simulink model "verify_com_acceleration_computation"  (R2015a)
settings: Solver=ode45  StartTime=0.0  StopTime=1.2  RelTol=1e-3
undefined symbols (not defined in the file or in its folder): A_kalman_transverse, A_kalman_vertical, B_kalman_transverse, B_kalman_vertical, C_kalman_transverse, C_kalman_vertical, com_leg_motor, com_torso, Discrete, g, initial_dx_estimate, initial_dy_estimate, initial_dz_estimate, initial_z_estimate, kalman_stance_slip_threshold, lateral_offset, m_leg, m_leg_motor, m_torso, m_total_real, P0_kalman_transverse, P0_kalman_vertical, pelvis_to_imu, R_kalman_accelerometer, R_kalman_foot_slip, R_kalman_foot_stance, sample_time, Time, X, Y, Z
libraries: nesl_utility x121, sm_lib x43, simulink x3, ctrlSharedLib x3
(part 3 of 3)

== matlab function verify_com_acceleration_computation/Kalman Filtering/Measurement Noise Covariance Matricies ==
  data: R_transverse output; vertical_GRF_L input; vertical_GRF_R input; R_kalman_foot_stance parameter; R_kalman_foot_slip parameter; R_kalman_accelerometer parameter; sample_time parameter; m_total_real parameter; g parameter; R_vertical output; kalman_stance_slip_threshold parameter
function [R_transverse, R_vertical] =...
         MeasurementNoiseCovariance(vertical_GRF_L, vertical_GRF_R, ...
           R_kalman_foot_stance, R_kalman_foot_slip, R_kalman_accelerometer, sample_time, m_total_real, g, kalman_stance_slip_threshold)

    % filter states: [dx_w]; [dy_w]; [dz_w];
    % measurements:  [dx_w-dfL + dfL_hat; dx_w-dfR + dfR_hat]; 

    ratio_L = 1;%max(0, min(vertical_GRF_L/(kalman_stance_slip_threshold*m_total_real*g),1)); % ratio is 0 if no load, 1 if at least equilibrium
    ratio_R = 0;%max(0, min(vertical_GRF_R/(kalman_stance_slip_threshold*m_total_real*g),1));
    R_transverse = diag([ratio_L*R_kalman_foot_stance + (1-ratio_L)*R_kalman_foot_slip, ...
                         ratio_R*R_kalman_foot_stance + (1-ratio_R)*R_kalman_foot_slip, ...
                         R_kalman_accelerometer])/sample_time;
    R_vertical = diag([ratio_L*R_kalman_foot_stance  + (1-ratio_L)*R_kalman_foot_slip,...
                       ratio_R*R_kalman_foot_stance  + (1-ratio_R)*R_kalman_foot_slip,...
                       R_kalman_accelerometer])/sample_time;
end

== matlab function verify_com_acceleration_computation/Kalman Filtering/eigen values ==
  data: Z input; E output
function E = eigen(Z)
    E = real(eig(Z));
    E = sort(E);
end

== matlab function verify_com_acceleration_computation/Kalman Filtering/eigen values1 ==
  data: Z input; E output
function E = eigen(Z)
    E = real(eig(Z));
    E = sort(E);
end

== matlab function verify_com_acceleration_computation/Kalman Filtering/eigen values2 ==
  data: Z input; E output
function E = eigen(Z)
    E = real(eig(Z));
    E = sort(E);
end

== matlab function verify_com_acceleration_computation/Compute COM Translational Acceleration (IMU uses non-rotating measurement frame) ==
  data: torso_angular_velocities input; com_acceleration_yawed output; torso_angular_accelerations input; imu_translational_accelerations_body input; torso_roll input; torso_pitch input; hip_roll_accelerations input; right_hip_roll input; left_hip_roll input; pelvis_to_imu parameter; com_torso parameter; com_leg_motor parameter; g parameter; m_leg_motor parameter; m_leg parameter; m_torso parameter; torso_com_acceleration_world output; torso_com_relative_acceleration_world output; torso_com_relative_velocity_world output; imu_to_torso_com_world output; imu_acceleration_world output; right_hip_acceleration_world output; left_hip_acceleration_world output
function [com_acceleration_yawed,torso_com_acceleration_world,torso_com_relative_acceleration_world,...
          torso_com_relative_velocity_world, imu_to_torso_com_world,imu_acceleration_world,...
          right_hip_acceleration_world, left_hip_acceleration_world] = compute_com_acceleration(torso_angular_velocities, torso_angular_accelerations, imu_translational_accelerations_body, torso_roll, torso_pitch, hip_roll_accelerations, right_hip_roll, left_hip_roll, pelvis_to_imu, com_torso, com_leg_motor, g, m_leg_motor, m_leg, m_torso)

    % Body frame to Yawed world frame rotations  
    R_body_to_yawed = R_pitch(torso_pitch(1))*R_roll(torso_roll(1));
    dR_body_to_yawed = dR_pitch(torso_pitch(1),torso_pitch(2))*R_roll(torso_roll(1)) + R_pitch(torso_pitch(1))*dR_roll(torso_roll(1),torso_roll(2));
    ddR_body_to_yawed = ddR_pitch(torso_pitch(1),torso_pitch(2),torso_angular_accelerations(2))*R_roll(torso_roll(1)) ...
                        + R_pitch(torso_pitch(1))*ddR_roll(torso_roll(1),torso_roll(2),torso_angular_accelerations(1)) ... 
                        + 2*dR_pitch(torso_pitch(1),torso_pitch(2))*dR_roll(torso_roll(1),torso_roll(2));

    % Compute translational acceleration of torso COM    
    imu_to_torso_com_world = R_body_to_yawed*(com_torso - pelvis_to_imu)';
    torso_com_relative_velocity_world = cross(torso_angular_velocities, imu_to_torso_com_world);
    torso_com_relative_acceleration_world = cross(torso_angular_accelerations, imu_to_torso_com_world) + cross(torso_angular_velocities, torso_com_relative_velocity_world);
    imu_to_pelvis_world =  R_body_to_yawed*(-pelvis_to_imu)';
    imu_acceleration_world = R_body_to_yawed*imu_translational_accelerations_body;
    torso_com_acceleration_world = imu_acceleration_world + torso_com_relative_acceleration_world;
    
    % Compute accelerations of hip COMs
    R_right_hip_to_body =     R_roll(-pi/2+right_hip_roll(1));
    dR_right_hip_to_body =   dR_roll(-pi/2+right_hip_roll(1), right_hip_roll(2));
    ddR_right_hip_to_body = ddR_roll(-pi/2+right_hip_roll(1), right_hip_roll(2), hip_roll_accelerations(1));
    R_left_hip_to_body =     R_roll(pi/2-left_hip_roll(1));
    dR_left_hip_to_body =   dR_roll(pi/2-left_hip_roll(1), -left_hip_roll(2));
    ddR_left_hip_to_body = ddR_roll(pi/2-left_hip_roll(1), -left_hip_roll(2), -hip_roll_accelerations(2));
    
    pelvis_relative_acceleration_world = cross(torso_angular_accelerations, imu_to_pelvis_world) + cross(torso_angular_velocities, cross(torso_angular_velocities, imu_to_pelvis_world));
    pelvis_acceleration_world = imu_acceleration_world + pelvis_relative_acceleration_world;    
    
    left_hip_acceleration_world = pelvis_acceleration_world + (ddR_body_to_yawed*R_left_hip_to_body + 2*(dR_body_to_yawed*dR_left_hip_to_body) + R_body_to_yawed*ddR_left_hip_to_body)*com_leg_motor';
    right_hip_acceleration_world = pelvis_acceleration_world + (ddR_body_to_yawed*R_right_hip_to_body + 2*(dR_body_to_yawed*dR_right_hip_to_body) + R_body_to_yawed*ddR_right_hip_to_body)*(com_leg_motor.*[1,-1,1])';
    
    % Compute total system COM acceleration
    m_hip = m_leg+m_leg_motor;
    m_total = 2*m_hip + m_torso;
    com_acceleration_yawed = (m_torso*torso_com_acceleration_world + m_hip*(left_hip_acceleration_world + right_hip_acceleration_world))/m_total;
     
    
    %com_acceleration_yawed(3) = com_acceleration_yawed(3) - g; % used on real system
    
end

function R_yp = R_pitch(theta) % map from pitched to yawed
  R_yp = [cos(theta), 0, sin(theta); ...
          0, 1, 0; ...
          -sin(theta), 0, cos(theta)];
end
function dR_yp = dR_pitch(theta,dtheta)
  dR_yp = dtheta*[-sin(theta), 0, cos(theta); ...
                  0, 0, 0; ... 
                  -cos(theta), 0, -sin(theta)];
end
function ddR_yp = ddR_pitch(theta,dtheta,ddtheta)
  ddR_yp = ddtheta*[-sin(theta), 0, cos(theta); ...
                    0, 0, 0; ... 
                    -cos(theta), 0, -sin(theta)] ...
           + dtheta^2*[-cos(theta), 0, -sin(theta); ...
                     0, 0, 0; ...
                     sin(theta), 0, -cos(theta)];
end
function R_pr = R_roll(phi) % map from rolled to pitched
  R_pr = [1, 0, 0; ...
          0, cos(phi), -sin(phi); ...
          0, sin(phi), cos(phi)]; 
end
function dR_pr = dR_roll(phi,dphi)
  dR_pr = dphi*[0, 0, 0; ...
                0, -sin(phi), -cos(phi); ...
                0, cos(phi), -sin(phi)];
end
function ddR_pr = ddR_roll(phi, dphi, ddphi)
  ddR_pr = ddphi*[0, 0, 0; ...
                  0, -sin(phi), -cos(phi); ...
                  0, cos(phi), -sin(phi)] ...
           + dphi^2*[0, 0, 0; ...
                   0, -cos(phi), sin(phi);...
                   0, -sin(phi), -cos(phi)];
end

== matlab function verify_com_acceleration_computation/PositionUsingRobotGeometry ==
  data: roll input; pitch input; yaw input; left_leg_lateral_angle input; right_leg_lateral_angle input; m_torso parameter; m_leg_motor parameter; m_leg parameter; com_torso parameter; com_leg_motor parameter; lateral_offset parameter; com_pelvis output; dcom_pelvis output
% Returns 2D COM relative to primary foot
function [com_pelvis, dcom_pelvis] = ...
         ComPositionUsingRobotGeometry( roll, pitch, yaw, ...
                                    left_leg_lateral_angle, ...
                                    right_leg_lateral_angle, ...
                                    m_torso, m_leg_motor, m_leg, com_torso, com_leg_motor, lateral_offset)
                    
    q =  [roll(1), pitch(1), yaw(1), 0, left_leg_lateral_angle(1), 0, 0, right_leg_lateral_angle(1), 0];
    dq = [roll(2), pitch(2), yaw(2), 0, left_leg_lateral_angle(2), 0, 0, right_leg_lateral_angle(2), 0];
                    
    [ com_pelvis, dcom_pelvis, ...
      ~, ~, ...
      ~, ~ ] = ...
    ComCalculationFromRobot( q, dq, m_torso, m_leg_motor, m_leg, com_torso, com_leg_motor, lateral_offset );


end
